simulink model "SHEV_Camaro_PwrLossMdl"  (R2018b)
settings: Solver=ode2  StartTime=0.0  StopTime=simDrv.time_s(end)  FixedStep=t_step  RelTol=1e-3
values from neighbouring files (symbols this model uses):
  A123_ESS =     [PwrLossMdl_A123Battery.mat]
  adj_motEffMap = [0.25 0.31 0.37 0.38 0.4 0.49 0.58 0.64 0.31 0.36 0.39 0.406 ... (72 elements, 8x9)]    [PwrLossMdl_PropSysEffData.mat]
  adjbsfc_map = [1051 1388 1174 1085 895 602 501 388 388 1051 1134 996 ... (81 elements, 9x9)]    [PwrLossMdl_GenSysEffData.mat]
  adjbsfc_spdbpt = [4003 4510 4987 5412 5800 5986 6322 6643 6889]    [PwrLossMdl_GenSysEffData.mat]
  adjbsfc_trqbpt = [10 15 20 25 30 35 40 45 50]    [PwrLossMdl_GenSysEffData.mat]
  C1 = [20000 20000 46318.5184323 46009.1793978 1021.23087801 1108.29786665 9922.48088723 10264.7269718 18293.5148586 29962.1621632 36298.3673472 37544.2700719 ... (41 elements, 1x41)]    [PwrLossMdl_ESS.mat]
  C2 = [20000 20000 46318.5184106 46009.1793608 1021.23035996 1108.29602087 9922.4809203 10264.72697 18293.5148606 29962.1621637 36298.3673482 37544.2700716 ... (41 elements, 1x41)]    [PwrLossMdl_ESS.mat]
  contMotTrq = [250 250 250 250 250 250 225 190 170]    [PwrLossMdl_PropSysEffData.mat]    (also in startPwrLossMdl.m = [180;180;180;180;180;180;180;180;170])
  cs_ll = 0.15    [startPwrLossMdl.m]
  cs_ul = 0.25    [startPwrLossMdl.m]
  E85_LHV = 30000    [startPwrLossMdl.m]
  mot_gbx_rat = 4.2    [startPwrLossMdl.m]
  motSpdVec = [1 500 1000 1500 2000 2500 3000 3500 4000]    [PwrLossMdl_PropSysEffData.mat]
  motTrqVec = [1 25 50 75 100 125 150 175]    [PwrLossMdl_PropSysEffData.mat]
  R0 = [0.5 0.5 0.413858741447 0.181330616185 0.123924684061 0.082623865753 0.114591066521 0.096554690516 0.0949331545326 0.124564294889 0.118490098825 0.107959033825 ... (41 elements, 1x41)]    [PwrLossMdl_ESS.mat]
  R1 = [0.5 0.5 0.513602817558 0.526624804767 0.484906164492 0.489343525408 0.493637128787 0.498122066152 0.500091294983 0.500054252951 0.500314275839 0.500483147312 ... (41 elements, 1x41)]    [PwrLossMdl_ESS.mat]
  R2 = [0.5 0.5 0.513602817535 0.526624804695 0.484906164494 0.489343525401 0.493637128787 0.498122066152 0.500091294984 0.50005425295 0.500314275838 0.500483147311 ... (41 elements, 1x41)]    [PwrLossMdl_ESS.mat]
  rho_fuel_gpL = 783    [startPwrLossMdl.m]
  simDrv = EEC_Single    [startPwrLossMdl.m]
  soc_bpt = [0 0.025 0.05 0.075 0.1 0.125 0.15 0.175 0.2 0.225 0.25 0.275 ... (41 elements, 1x41)]    [PwrLossMdl_ESS.mat]
  t_step = 0.1    [startPwrLossMdl.m]
  tire_rad_m = 0.346    [startPwrLossMdl.m]
  V_fuel_init_gal = 7    [startPwrLossMdl.m]
undefined symbols (not defined in the file or in its folder): DiscIntNeverNeededParam, N_OptResults, OptResults
libraries: simulink x10, custom_func x2, dspstat3 x1
(part 2 of 2)

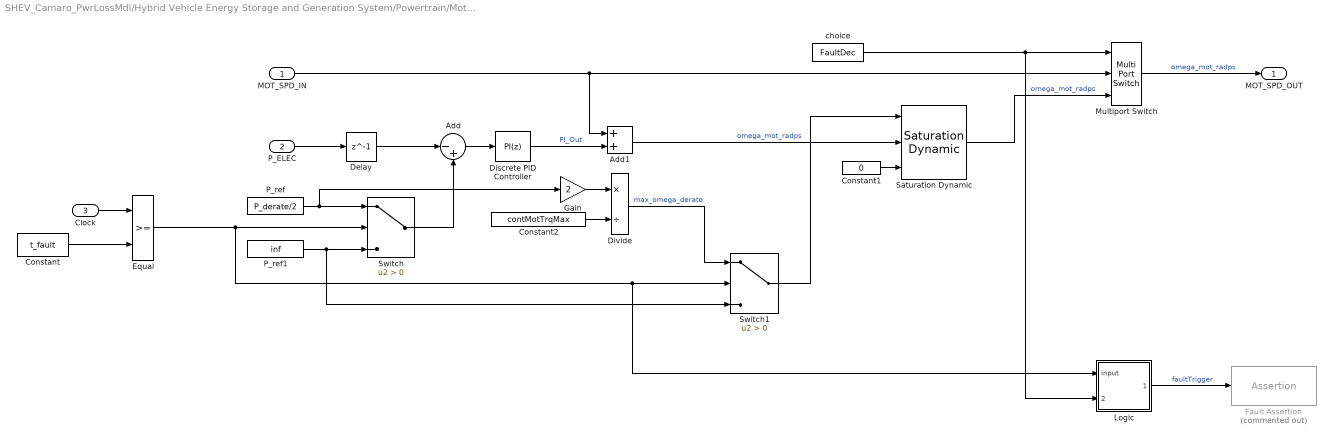
== system SHEV_Camaro_PwrLossMdl/Hybrid Vehicle Energy Storage and Generation System/Powertrain/Motor Fault Injection ==
  MOT_SPD_IN : Inport
  P_ELEC : Inport  Port=2
  Clock : Inport  Port=3
  Add : Sum  Inputs=|-+
  Add1 : Sum
  Constant : Constant  Value=t_fault
  Constant1 : Constant  Value=0
  Constant2 : Constant  Value=contMotTrqMax
  Delay : Delay  DelayLength=1
  Discrete PID Controller : simulink/Continuous/PID Controller  Controller=PI  Form=Parallel  TimeDomain=Discrete-time  SampleTime=-1  IntegratorMethod=Forward Euler  FilterMethod=Forward Euler  ControllerParametersSource=internal  P=0.002  I=0.003  D=0  UseFilter=on  N=100  TunerSelectOption=Transfer Function Based (PID Tuner App)  InitialConditionSource=internal  InitialConditionForIntegrator=0  InitialConditionForFilter=0  DifferentiatorICPrevScaledInput=0  ExternalReset=none  TrackingMode=off  Kt=1  LimitOutput=on  UpperSaturationLimit=0  LowerSaturationLimit=-inf  LinearizeAsGain=off  AntiWindupMode=clamping  Kb=1  POutMin=[]  POutMax=[]  IOutMin=[]  IOutMax=[]  DOutMin=[]  DOutMax=[]  NOutMin=[]  NOutMax=[]  SumOutMin=[]  SumOutMax=[]  SaturationOutMin=[]  SaturationOutMax=[]  PParamMin=[]  PParamMax=[]  IParamMin=[]  IParamMax=[]  DParamMin=[]  DParamMax=[]  NParamMin=[]  NParamMax=[]  KbParamMin=[]  KbParamMax=[]  KtParamMin=[]  KtParamMax=[]  KbOutMin=[]  KbOutMax=[]  KtOutMin=[]  KtOutMax=[]  IntegratorOutMin=[]  IntegratorOutMax=[]  FilterOutMin=[]  FilterOutMax=[]  SumI1OutMin=[]  SumI1OutMax=[]  SumI2OutMin=[]  SumI2OutMax=[]  SumI3OutMin=[]  SumI3OutMax=[]  SumI4OutMin=[]  SumI4OutMax=[]  SumDOutMin=[]  SumDOutMax=[]  DifferentiatorOutMin=[]  DifferentiatorOutMax=[]  FilterDiffOutCoefMin=[]  FilterDiffOutCoefMax=[]  ReciprocalOutMin=[]  ReciprocalOutMax=[]  SumDenOutMin=[]  SumDenOutMax=[]  SumNumOutMin=[]  SumNumOutMax=[]  DivideOutMin=[]  DivideOutMax=[]  IntegratorContinuousStateAttributes=''  IntegratorStateMustResolveToSignalObject=off  IntegratorRTWStateStorageClass=Auto  FilterContinuousStateAttributes=''  FilterStateMustResolveToSignalObject=off  FilterRTWStateStorageClass=Auto  ParallelPVariant=InternalParameters  IdealPVariant=Disabled  IVariant=InternalParameters  DVariant=Disabled  IntegratorVariant=Discrete  SatVariant=Enabled  AWVariant=DiscClampingParallel  PCopyVariant=Disabled  TRVariant=Disabled  FdbkBlocksVariant=Forward  IdealPFdbkVariant=Disabled  SatFdbkVariant=Disabled  DerivativeFilterVariant=Disabled  NVariant=Disabled  NCopyVariant=Disabled_SignalSpec  FilterICVariant=Disabled  IntegratorICVariant=InternalICs  ExternalResetVariant=Disabled  TRSumVariant=Passthrough  SumFdbkVariant=Disabled  SumVariant=Sum_PI
  Divide : Product  Inputs=*/
  Equal : RelationalOperator  OutDataTypeStr=boolean  RndMeth=Simplest
  Fault Assertion : Assertion  Commented=on  AssertionFailFcn=|  StopWhenAssertionFail=off
      | set_param(bdroot,'SimulationCommand','pause');
      | disp('## Paused due to Motor fault insertion')
  Gain : Gain  Gain=2
  Logic : Stateflow chart  TreatAsAtomicUnit=on
  Multiport Switch : MultiPortSwitch  DataPortOrder=Zero-based contiguous  Inputs=2  zeroidx=on
  P_ref : Constant  Value=P_derate/2
  P_ref1 : Constant  Value=inf
  Saturation Dynamic : simulink/Discontinuities/Saturation Dynamic  OutMin=[]  OutMax=[]  OutDataTypeStr=Inherit: Same as second input  OutDataType=fixdt(1, 16)  OutScaling=2^-10  DoSatur=off
  Switch : Switch  Criteria=u2 > Threshold
  Switch1 : Switch  Criteria=u2 > Threshold
  choice : Constant  Value=FaultDec
  MOT_SPD_OUT : Outport
  wires:
  Multiport Switch/1 -> MOT_SPD_OUT/1  "omega_mot_radps"
  choice/1 -> Logic/2(choice), Multiport Switch/1
  Add/1 -> Discrete PID Controller/1
  P_ELEC/1 -> Delay/1
  Delay/1 -> Add/1
  Discrete PID Controller/1 -> Add1/2  "PI_Out"
  MOT_SPD_IN/1 -> Multiport Switch/2, Add1/1
  P_ref/1 -> Gain/1, Switch/1
  Saturation Dynamic/1 -> Multiport Switch/3  "omega_mot_radps"
  Add1/1 -> Saturation Dynamic/2  "omega_mot_radps"
  Clock/1 -> Equal/1
  Constant/1 -> Equal/2
  Equal/1 -> Logic/1(input), Switch1/2, Switch/2
  Switch/1 -> Add/2
  P_ref1/1 -> Switch1/3, Switch/3
  Constant1/1 -> Saturation Dynamic/3
  Gain/1 -> Divide/1
  Constant2/1 -> Divide/2
  Divide/1 -> Switch1/1  "max_omega_derate"
  Switch1/1 -> Saturation Dynamic/1
  Logic/1(trigger) -> Fault Assertion/1  "faultTrigger"

== matlab function SHEV_Camaro_PwrLossMdl/Hybrid Vehicle Energy Storage and Generation System/Powertrain/MATLAB Function ==
  data: v_veh_mps input; v_veh_out_mps output; flag output
function [v_veh_out_mps,flag] = zerocheck(v_veh_mps)
    % Checks if the input speed is zero. 
    % If zero: sets the flag = 1, to change torque value to zero.
    % If not zero: sets the flag = 0, no change to the the torque value.
    
    if v_veh_mps == 0
        flag = 1;
        v_veh_out_mps = v_veh_mps;
    else
        flag = 0;
        v_veh_out_mps = v_veh_mps;
    end
end

== matlab function SHEV_Camaro_PwrLossMdl/Hybrid Vehicle Energy Storage and Generation System/MATLAB Function ==
  data: inp input; out output
function out = addnoise(inp)
snr = 25;

out = awgn(inp,snr,'measured');

== matlab function SHEV_Camaro_PwrLossMdl/Vehicle 2DOF Longitudinal and Pitch Model/Vehicle Dynamics Model 2 DOF (Longitudinal and Pitch) ==
  data: v_spd input; P_veh output; rg_pct input; dt input; Trq_dem output; acc_veh output; KE_veh output; Pwr_RR output; Pwr_Load output; dist_m output; elev_m output
function [P_veh, Trq_dem, acc_veh, KE_veh, Pwr_RR, Pwr_Load, dist_m, elev_m] = vehdyn2dof(v_spd,rg_pct,dt)
    % DESCRIPTION: The 2DOF Longitudinal and Pitch Model for the vehicle
    % uses the longitudinal road load equation comprising of Aerodynamic
    % Resistance, Climbing Resistance, Rolling Resistance as resistive
    % forces on the vehicle.
    %
    % F_veh [N] = F_trac + F_ar + F_cr + F_rr;  --------- (1)
    % P_veh [W] = F_veh [N] * v_veh [m/s];      --------- (2)
    %
    % Note: Pitch dynamics will be added to the model once COG height for
    % the car is determined. Currently only 1DOF longitudinal dynamics
    % exist.
    
    %% Pre-processing
    persistent v_spd_old dist elev
    if isempty(v_spd_old) && isempty(dist) && isempty(elev)
        v_spd_old = v_spd;
        dist = 0;
        elev = 0;
        flag = 1;
    else
        flag = 0;
    end
    alpha = atan(rg_pct/100);
    
    %% Static Parameters
    % -- Vehicle
    A_veh = 0.4;        % [m^2]
    C_d = 0.34;         % drag coefficient [-]
    m_veh = 2012;       %1875;       % [kg]
    P_tire = 32;        % [psi]
    R_tire = 0.346;     % [m]
    N_drvnWhl = 2;      % [-]
    Rat_gbx = 4.2;
    
    % -- Environment
    g = 9.81;           % acceleration due to gravity [m/s^2]
    rho_air = 1.225;    % STP density [kg/m^3]
    
    %% Dynamic Parameters
    C_rr = 0.005 + ((0.06895/P_tire) * ...
        (0.01 + (0.0095 * ((2.778 * (10^-3) * v_spd)^2))));            
    % function of tire pressure and vehicle speed [psi, mps]
    
    %% Vehicle Power Calculation
    if flag == 1
        P_veh = 0;
        Trq_dem = 0; 
        acc_veh = 0;
        KE_veh = 0;
        Pwr_RR = 0;
        Pwr_Load = 0;
        dist_m = dist;
        elev_m = elev;
    else
        acc_veh = (v_spd - v_spd_old)/dt;
        P_veh = ((m_veh * acc_veh) + ...
            (0.5 * rho_air * A_veh * C_d * (v_spd ^ 2)) + ...
            (m_veh * g * sin(alpha)) + ...
            (C_rr * m_veh * g)) * (v_spd);
        Trq_dem = ((P_veh/v_spd) * R_tire)/((N_drvnWhl * Rat_gbx));
        KE_veh = 0.5 * m_veh * ((v_spd^2) - (v_spd_old^2));
        dist_del = (v_spd_old * dt) + (0.5 * acc_veh * (dt^2));
        dist = dist + dist_del;
        elev = elev + ((rg_pct/100)*dist_del);
        dist_m = dist;
        elev_m = elev;
        v_spd_old = v_spd;
        Pwr_RR = (C_rr * m_veh * g) * (v_spd);
        Pwr_Load = ((0.5 * rho_air * A_veh * C_d * (v_spd ^ 2)) + ...
            (m_veh * g * sin(alpha)) + ...
            (C_rr * m_veh * g)) * (v_spd);
    end
    
end

== stateflow chart SHEV_Camaro_PwrLossMdl/Hybrid Vehicle Energy Management Control/Regen Braking Algorithm ==
  note: %P_reg_W
  state NoBraking
    du:
    P_reg_W = 0;
    P_mechbrk_W = 0;
    P_batt_W = P_elec_W;
  state Braking
    state RegenDisabled
      du:
      P_reg_W = 0;
      P_mechbrk_W = P_elec_W;
      P_batt_W = 0;
    state RegenEnabled
      state LightBraking
        du:
        P_reg_W = P_elec_W;
        P_mechbrk_W = P_elec_W - P_reg_W;
        P_batt_W = P_reg_W;
      state HeavyBraking
        du:
        P_reg_W = P_motreg_max_W;
        P_mechbrk_W = P_elec_W - P_reg_W;
        P_batt_W = P_reg_W;
      (default) -> LightBraking
      LightBraking -> HeavyBraking : [P_elec_W <= ...
          | P_motreg_max_W]
      HeavyBraking -> LightBraking : [P_elec_W >= ...
          | P_motreg_max_W]
    (default) -> RegenDisabled
    RegenDisabled -> RegenEnabled : [SoC <= 0.95]
    RegenEnabled -> RegenDisabled : [SoC > 0.95]
  (default) -> NoBraking
  NoBraking -> Braking : [P_elec_W < 0]
  Braking -> NoBraking : [P_elec_W >= 0]
  data: P_elec_W input; P_motreg_max_W input; P_mechbrk_W output double; P_batt_W output double; P_reg_W local double; SoC input

== stateflow chart SHEV_Camaro_PwrLossMdl/Hybrid Vehicle Energy Storage and Generation System/Battery EPO Logic/Battery EPO Constraint Logic ==
  state NoEPO
    du:
    epo_flag = 0;
  state EPO
    du:
    epo_flag = 1;
  (default) -> NoEPO
  NoEPO -> EPO : [LoadCurr < DchgCurrLim]
  EPO -> NoEPO : [LoadCurr >= DchgCurrLim]
  data: DchgCurrLim input; LoadCurr input; epo_flag output double

== stateflow chart SHEV_Camaro_PwrLossMdl/Hybrid Vehicle Energy Management Control/Rule Based Algorithm - Standard/Rule-Based Energy Mode Control ==
  state Initialization
  state CDMode
    du:
    mode = 0;
    genstat = 0;
  state CSModeGen
    du:
    mode = 1;
    genstat = 1;
  state CSModeNoGen
    du:
    mode = 1;
    genstat = 0;
  (default) -> Initialization
  Initialization -> (junction 7) [order 1] : [batsoc_frac <= init_soc && ...
      | batsoc_frac >= cs_ll]
  Initialization -> (junction 10) [order 2] : [batsoc_frac < cs_ll]
  (junction 7) -> CDMode
  (junction 10) -> CSModeGen
  CDMode -> CSModeGen : [batsoc_frac < cs_ll]
  CSModeGen -> CSModeNoGen : [batsoc_frac >= cs_ul]
  CSModeNoGen -> CSModeGen : [batsoc_frac < cs_ll]
  data: batsoc_frac input; cs_ll input; cs_ul input; init_soc input; genstat output double; mode output double

== matlab function SHEV_Camaro_PwrLossMdl/Hybrid Vehicle Energy Management Control/Rule Based Algorithm - Standard/Variable Power Request ==
  data: VehSpd_kph input; PwrMode output
function PwrMode = VarPwrReq(VehSpd_kph)
    if VehSpd_kph >= 0 && VehSpd_kph < 48
        PwrMode = 0;
    elseif VehSpd_kph >= 48 && VehSpd_kph < 97
        PwrMode = 1;
    else
        PwrMode = 2;
    end
end

== matlab function SHEV_Camaro_PwrLossMdl/Hybrid Vehicle Energy Storage and Generation System/A123 ESS Model/OCV_Battery/OCV Function ==
  data: soc input; ocv output; current input
function ocv = fcn(soc, current)

if current < 0
    %% 0-20 Model Fit
    if (soc <= 0.2)
        ocv = 3.17*exp(0.1*soc) - 2.76*exp(-65.25*soc);
    %% 20-80 Model Fit
    elseif (soc > 0.2 && soc <= 0.8)
        ocv = 0.155*soc + 3.2;
        % ocv = 0.165*soc + 3.20; OG
    %% 80-100 Model Fit
    else
        ocv = 0.2*(soc^74.2) + 3.33;
    end
else
    %% 0-20 Model Fit
    if (soc <= 0.2)
        ocv = 3.19*exp(0.098*soc) - 1.09*exp(-48.81*soc);
    %% 20-80 Model Fit
    elseif (soc > 0.2 && soc <= 0.8)
        ocv = 0.148*soc + 3.2;
        % ocv = 0.148*soc + 3.222;
    %% 80-100 Model Fit
    else
        ocv = 0.336*(soc^108.2) + 3.34;
    end
end

== stateflow chart SHEV_Camaro_PwrLossMdl/Hybrid Vehicle Energy Management Control/Proposed ReOpt DP Algorithm/Wait ==
  state Initialization
    en:
    Counter = 0;
    Trigger = 1;
  state InState
    du:
    Trigger = 1;
  state Wait1
  state Wait
  state OutState
    en:
    Trigger = 0;
    du:
    Trigger = 1;
    ex:
    Trigger = 1;
  (default) -> Initialization
  Initialization -> InState
  Wait1 -> InState : after(5.0,sec)
  Wait -> InState [order 1] : [ReOptReq == 0]
  InState -> Wait : [ReOptReq == 1]
  OutState -> Wait1 : [ReOptReq == 0]
  Wait -> OutState [order 2] : after(5.0,sec){Counter = Counter + 1;}
  data: ReOptReq input; Trigger output double; Counter output double

== stateflow chart SHEV_Camaro_PwrLossMdl/Hybrid Vehicle Energy Management Control/REx Fault Insertion Subsystem/Logic ==
  state NoFault
    en:
    trigger = 1;
    du:
    trigger = 1;
  state Fault
    en:
    trigger = 0;
    du:
    trigger = 1;
  (default) -> NoFault
  NoFault -> Fault : [input1 == 0 ||...
      | input2 == 0]
  data: trigger output double; input1 input; input2 input

== matlab function SHEV_Camaro_PwrLossMdl/Hybrid Vehicle Energy Management Control/Proposed ReOpt DP Algorithm/Optimal Pgen Lookup ==
  data: index input; element output; vector input
function element = idxLookup(index,vector)
% idxLookup is a custom function that returns element corresponding to
% index in a 1-D vector.
element = vector(index);
end

== matlab function SHEV_Camaro_PwrLossMdl/Hybrid Vehicle Energy Management Control/Proposed ReOpt DP Algorithm/Optimal SoC Lookup ==
  data: index input; element output; vector input
function element = idxLookup(index,vector)
% idxLookup is a custom function that returns element corresponding to
% index in a 1-D vector.
element = vector(index);
end

== matlab function SHEV_Camaro_PwrLossMdl/Hybrid Vehicle Energy Management Control/Proposed ReOpt DP Algorithm/Optimal EC_Wh_m ==
  data: index input; element output; vector input
function element = idxLookup(index,vector)
% idxLookup is a custom function that returns element corresponding to
% index in a 1-D vector.
element = vector(index);
end

== stateflow chart SHEV_Camaro_PwrLossMdl/Hybrid Vehicle Energy Storage and Generation System/Powertrain/Motor Fault Injection/Logic ==
  state NoFault
    en:
    trigger = 1;
    du:
    trigger = 1;
  state Fault
    en:
    trigger = 0;
    du:
    trigger = 1;
  (default) -> NoFault
  NoFault -> Fault : [input == 1 && ...
      | choice == 1]
  data: trigger output double; input input; choice input

== matlab function SHEV_Camaro_PwrLossMdl/Hybrid Vehicle Energy Management Control/EREV EM Custom MPC/Custom SOC MPC ==
  data: x_soc_k input; u_soc_ref_vec input size=[30 1]; x_soc_est_k_1 output size=[30 1] [0..1]; u_Paux_k_1 input; u_P_gen_k_1 input; u_est_spd_vec input size=[30 1]; u_est_acc_vec input size=[30 1]; md_grade_vec input size=[30 1]; estHorizon input; ctlHorizon input; Ts input; P_gen_opt output size=[30 1]; SOC_opt output size=[30 1]; status output; p output
function [x_soc_est_k_1,P_gen_opt,SOC_opt,status,p]  = soc_mpc(x_soc_k,u_soc_ref_vec,u_Paux_k_1,u_P_gen_k_1,u_est_spd_vec,u_est_acc_vec,md_grade_vec,estHorizon,ctlHorizon,Ts)
% ,b,H,f,A
%% Linearized Vehicle Power Model - UW EREV
m = 2012;
g = 9.81;
% Aerodynamic Drag Resistance Power Coefficient
Af = 0.4;
Cd = 0.34;
rho = 1.225;
A1 = 0.5 * Af * Cd * rho;
% Rolling Resistance Power Coefficient
Cr = 0.00502;
B1 = m * g * Cr;
% Climbing Resistance Power Coefficient
C1 = m * g;
% Battery information
Ebatt = 18900;

%% Estimation vector 
persistent soc_est_vec
if isempty(soc_est_vec)
    soc_est_vec = ones([estHorizon 1]);
end

%% Model based estimation
Pbatt = zeros([estHorizon 1]);
for k = 1:estHorizon
    Pbatt(k,1) = u_Paux_k_1 - u_P_gen_k_1 + (m * u_est_spd_vec(k,1) * u_est_acc_vec(k,1))...
            + (A1 * (u_est_spd_vec(k,1)^3)) + (B1 * u_est_spd_vec(k,1))...
            + (C1 * (md_grade_vec(k,1)/100) * u_est_spd_vec(k,1));
    if Pbatt(k,1) < -15000
        Pbatt(k,1) = -15000;
    end
    if k == 1
        soc_est_vec(k,1) = x_soc_k - ((Ts/(Ebatt * 3600)) * Pbatt(k,1));
    else
        soc_est_vec(k,1) = soc_est_vec(k-1,1) - ((Ts/(Ebatt * 3600)) * Pbatt(k,1));
    end
end
x_soc_est_k_1 = soc_est_vec;
%% Optimal Generator Power - mpcqpActiveSetSolver
p1 = 1;
p2 = 1e8;
k1 = 0.000141 * Ts;  % g/W; %Ts/(3600*18900);    
k2 = 1;
H = eye(ctlHorizon * 3);
for j = 1:(ctlHorizon * 3)  
    if mod(j,3) == 1
        H(j,:) = H(j,:) * (p1 * k1 * k1);
    elseif mod (j,3) == 2
        H(j,:) = H(j,:) * (p2 * k2 * k2);
    else
        H(j,:) = H(j,:) * p2 * (u_soc_ref_vec(j/3)^2);
    end
end
H = 2 * H;
[L,p] = chol(H,'lower');
Linv = inv(L);

f = zeros([ctlHorizon*3 1]);
f(2:3:end) = -2 * p2 * k2 * k2 * u_soc_ref_vec(1:ctlHorizon);

ineqVec_1 = [1 0 0;
            -1 0 0;
             0 1 0;
             0 -1 0];
ineqVec_3 = [1 0 0 1 0 0 1 0 0;
            -1 0 0 -1 0 0 -1 0 0;
             0 1 0 0 1 0 0 1 0;
             0 -1 0 0 -1 0 0 -1 0];
ineqVec_5 = [1 0 0 1 0 0 1 0 0 1 0 0 1 0 0;
            -1 0 0 -1 0 0 -1 0 0 -1 0 0 -1 0 0;
             0 1 0 0 1 0 0 1 0 0 1 0 0 1 0;
             0 -1 0 0 -1 0 0 -1 0 0 -1 0 0 -1 0];
ineqVec_10 = [1 0 0 1 0 0 1 0 0 1 0 0 1 0 0 1 0 0 1 0 0 1 0 0 1 0 0 1 0 0;
             -1 0 0 -1 0 0 -1 0 0 -1 0 0 -1 0 0 -1 0 0 -1 0 0 -1 0 0 -1 0 0 -1 0 0;
              0 1 0 0 1 0 0 1 0 0 1 0 0 1 0 0 1 0 0 1 0 0 1 0 0 1 0 0 1 0;
              0 -1 0 0 -1 0 0 -1 0 0 -1 0 0 -1 0 0 -1 0 0 -1 0 0 -1 0 0 -1 0 0 -1 0];
ineqVec_15 = [ineqVec_5 ineqVec_10];
ineqVec_20 = [ineqVec_10 ineqVec_10];
ineqVec_25 = [ineqVec_5 ineqVec_20];
ineqVec_30 = [ineqVec_15 ineqVec_15];
switch ctlHorizon
    case 1
        mult = 1;
        A = ineqVec_1;
        b = [0 * mult; -15000 * mult; sum(x_soc_est_k_1(1:mult,1)); -(sum(x_soc_est_k_1(1:mult,1)) + (((15000 * Ts)/(18900 * 3600))*mult))];
        Aeq = [-(Ts/(18900 * 3600)) 1 0];
        beq = sum(x_soc_est_k_1(1:mult,1));
    case 3
        mult = 3;
        A = ineqVec_3;
        b = [0 * mult; -15000 * mult; sum(x_soc_est_k_1(1:mult,1)); -(sum(x_soc_est_k_1(1:mult,1)) + (((15000 * Ts)/(18900 * 3600))*mult))];
        tmp_Aeq = [-(Ts/(18900 * 3600)) 1 0];
        Aeq = [tmp_Aeq tmp_Aeq tmp_Aeq];
        beq = sum(x_soc_est_k_1(1:mult,1));
    case 5
        mult = 5;
        A = ineqVec_5;
        b = [0 * mult; -15000 * mult; sum(x_soc_est_k_1(1:mult,1)); -(sum(x_soc_est_k_1(1:mult,1)) + (((15000 * Ts)/(18900 * 3600))*mult))];
        tmp_Aeq = [-(Ts/(18900 * 3600)) 1 0];
        Aeq = [tmp_Aeq tmp_Aeq tmp_Aeq tmp_Aeq tmp_Aeq];
        beq = sum(x_soc_est_k_1(1:mult,1));
    case 10
        mult = 10;
        A = ineqVec_10;
        b = [0 * mult; -15000 * mult; sum(x_soc_est_k_1(1:mult,1)); -(sum(x_soc_est_k_1(1:mult,1)) + (((15000 * Ts)/(18900 * 3600))*mult))];
        tmp_Aeq = [-(Ts/(18900 * 3600)) 1 0];
        Aeq = [tmp_Aeq tmp_Aeq tmp_Aeq tmp_Aeq tmp_Aeq tmp_Aeq tmp_Aeq tmp_Aeq tmp_Aeq tmp_Aeq];
        beq = sum(x_soc_est_k_1(1:mult,1));
    case 15
        mult = 15;
        A = ineqVec_15;
        b = [0 * mult; -15000 * mult; sum(x_soc_est_k_1(1:mult,1)); -(sum(x_soc_est_k_1(1:mult,1)) + (((15000 * Ts)/(18900 * 3600))*mult))];
        tmp_Aeq = [-(Ts/(18900 * 3600)) 1 0];
        Aeq = [tmp_Aeq tmp_Aeq tmp_Aeq tmp_Aeq tmp_Aeq tmp_Aeq tmp_Aeq tmp_Aeq tmp_Aeq tmp_Aeq tmp_Aeq tmp_Aeq tmp_Aeq tmp_Aeq tmp_Aeq];
        beq = sum(x_soc_est_k_1(1:mult,1));
    case 20
        mult = 20;
        A = ineqVec_20;
        b = [0 * mult; -15000 * mult; sum(x_soc_est_k_1(1:mult,1)); -(sum(x_soc_est_k_1(1:mult,1)) + (((15000 * Ts)/(18900 * 3600))*mult))];
        tmp_Aeq = [-(Ts/(18900 * 3600)) 1 0];
        Aeq = [tmp_Aeq tmp_Aeq tmp_Aeq tmp_Aeq tmp_Aeq tmp_Aeq tmp_Aeq tmp_Aeq tmp_Aeq tmp_Aeq tmp_Aeq tmp_Aeq tmp_Aeq tmp_Aeq tmp_Aeq tmp_Aeq tmp_Aeq tmp_Aeq tmp_Aeq tmp_Aeq];
        beq = sum(x_soc_est_k_1(1:mult,1));
    case 25
        mult = 25;
        A = ineqVec_25;
        b = [0 * mult; -15000 * mult; sum(x_soc_est_k_1(1:mult,1)); -(sum(x_soc_est_k_1(1:mult,1)) + (((15000 * Ts)/(18900 * 3600))*mult))];
        tmp_Aeq = [-(Ts/(18900 * 3600)) 1 0];
        Aeq = [tmp_Aeq tmp_Aeq tmp_Aeq tmp_Aeq tmp_Aeq tmp_Aeq tmp_Aeq tmp_Aeq tmp_Aeq tmp_Aeq tmp_Aeq tmp_Aeq tmp_Aeq tmp_Aeq tmp_Aeq tmp_Aeq tmp_Aeq tmp_Aeq tmp_Aeq tmp_Aeq tmp_Aeq tmp_Aeq tmp_Aeq tmp_Aeq tmp_Aeq];
        beq = sum(x_soc_est_k_1(1:mult,1));
    case 30
        mult = 30;
        A = ineqVec_30;
        b = [0 * mult; -15000 * mult; sum(x_soc_est_k_1(1:mult,1)); -(sum(x_soc_est_k_1(1:mult,1)) + (((15000 * Ts)/(18900 * 3600))*mult))];
        tmp_Aeq = [-(Ts/(18900 * 3600)) 1 0];
        Aeq = [tmp_Aeq tmp_Aeq tmp_Aeq tmp_Aeq tmp_Aeq tmp_Aeq tmp_Aeq tmp_Aeq tmp_Aeq tmp_Aeq tmp_Aeq tmp_Aeq tmp_Aeq tmp_Aeq tmp_Aeq tmp_Aeq tmp_Aeq tmp_Aeq tmp_Aeq tmp_Aeq tmp_Aeq tmp_Aeq tmp_Aeq tmp_Aeq tmp_Aeq tmp_Aeq tmp_Aeq tmp_Aeq tmp_Aeq tmp_Aeq];
        beq = sum(x_soc_est_k_1(1:mult,1));
    otherwise
        mult = 30;
        A = ineqVec_30;
        b = [0 * mult; -15000 * mult; sum(x_soc_est_k_1(1:mult,1)); -(sum(x_soc_est_k_1(1:mult,1)) + (((15000 * Ts)/(18900 * 3600))*mult))];
        tmp_Aeq = [-(Ts/(18900 * 3600)) 1 0];
        Aeq = [tmp_Aeq tmp_Aeq tmp_Aeq tmp_Aeq tmp_Aeq tmp_Aeq tmp_Aeq tmp_Aeq tmp_Aeq tmp_Aeq tmp_Aeq tmp_Aeq tmp_Aeq tmp_Aeq tmp_Aeq tmp_Aeq tmp_Aeq tmp_Aeq tmp_Aeq tmp_Aeq tmp_Aeq tmp_Aeq tmp_Aeq tmp_Aeq tmp_Aeq tmp_Aeq tmp_Aeq tmp_Aeq tmp_Aeq tmp_Aeq];
        beq = sum(x_soc_est_k_1(1:mult,1));
end

opt = mpcqpsolverOptions;

iA0 = false(size(b));

[x,status] = mpcqpsolver(Linv,f,A,b,Aeq,beq,iA0,opt);
P_gen_opt = x(1:3:end);
SOC_opt = x(2:3:end);
end

== matlab function SHEV_Camaro_PwrLossMdl/Hybrid Vehicle Energy Management Control/Prediction Vector Generator/Kinematic State Predictor ==
  data: inpvec_dist_m output size=[30 1]; vehSpd_mps input; vehAcc_mps2 input; distTrvld_m input; inpvec_vehSpd_mps output size=[30 1]; inpvec_vehAcc_ms2 output size=[30 1]; est_horizon_samples input; Ts input
function [inpvec_dist_m, inpvec_vehSpd_mps, inpvec_vehAcc_ms2]...
    = genkinest(vehSpd_mps, vehAcc_mps2, distTrvld_m, est_horizon_samples, Ts)

persistent v_old
if isempty(v_old)
    v_old = vehSpd_mps;
end

% Calculate vehicle acceleration at current time
veh_acc = vehAcc_mps2;

% Generate kinematic prediction vectors for est_horizon_samples
% The estimation horizon samples are based on 1 second time step
N = est_horizon_samples;
%% Linear Estimation - Not that good
% 1. Vehicle speed estimate for N (1 second) steps:
u = ones([N 1]) * vehSpd_mps;
a = eye(N) * veh_acc;
t = 1:1:N;
% --  Clamping values
tmp_vehSpd = u + (a*t');
tmp_vehAcc = diag(a);
tmp_vehAcc(tmp_vehSpd > 35.76) = 0;
tmp_vehAcc(tmp_vehSpd < 0) = 0;
tmp_vehSpd(tmp_vehSpd > 35.76) = 35.76;
tmp_vehSpd(tmp_vehSpd < 0) = 0;
inpvec_vehSpd_mps  = tmp_vehSpd;
inpvec_vehAcc_ms2 = tmp_vehAcc;

% 2. Vehicle distance estimate for N (1 second) steps:
uu = ones([N 1]) * vehSpd_mps;
temp_dist_m = (uu .* t') + (0.5 * tmp_vehAcc .* (t'.^2));
temp_dist_m(temp_dist_m < 0) = 0;
inpvec_dist_m = temp_dist_m + distTrvld_m;  % 

%% Speed limited - Exponential function estimation
% The upper and lower bounds on speed limit vary the acceleration values
% throughout the estimation horizon
% LL_SPD = 0;         % 0 mph
% UL_SPD = 35.8;      % 80 mph
% 
% if veh_acc >= 0
%     b_coeff = (4.95/(UL_SPD - LL_SPD)) * vehSpd_mps + 0.05;
% else
%     b_coeff = -(4.95/(UL_SPD - LL_SPD)) * vehSpd_mps + 5;
% end
% 
% a_coeff = veh_acc*2;
% 
% t_range = 1:1:N;
% 
% u = ones([N 1]) * vehSpd_mps;
% 
% for i = 2:N
%     u(i,1) = u(i-1,1) + (a_coeff * exp(-b_coeff * t_range(i)));
% end
% 
% inpvec_vehSpd_mps = u;
% inpvec_vehAcc_ms2 = (a_coeff * exp(-b_coeff * t_range'));
% inpvec_dist_m = distTrvld_m + cumsum(inpvec_vehSpd_mps);
end

== matlab function SHEV_Camaro_PwrLossMdl/Hybrid Vehicle Energy Management Control/Prediction Vector Generator/Optimal SoC Lookup ==
  data: index input size=[30 1]; element output size=[30 1]; vector input
function element = idxLookup(index,vector)
% idxLookup is a custom function that returns element corresponding to
% index in a 1-D vector.
element = vector(index);
end

== matlab function SHEV_Camaro_PwrLossMdl/Hybrid Vehicle Energy Management Control/Prediction Vector Generator/Road Grade Lookup ==
  data: index input size=[30 1]; element output size=[30 1]; vector input
function element = idxLookup(index,vector)
% idxLookup is a custom function that returns element corresponding to
% index in a 1-D vector.
element = vector(index);
end

== matlab function SHEV_Camaro_PwrLossMdl/Hybrid Vehicle Energy Management Control/Prediction Vector Generator/Vectorized Index Finder ==
  data: inpVector input; idx output size=[30 1]; queryElement input size=[30 1]; OUTOFRANGE_FLAG output
% This is a custom function block designed to determine the index of a
% search element in the available vector.
%
% ------------ Made by: Aman V. Kalia -----------------------------------
% ------------ University of Washington, Seattle ------------------------
% ------------ Made on: 12/04/2019 --------------------------------------
%
% Features:
% 1. It also handles edge cases where a direct find doesn't result in an 
% output. 
% 2. It throws a warning flag if the query SoC is out of range. Helpful in
% retriggering a recalculation.

function [idx,OUTOFRANGE_FLAG] = findidx(inpVector,queryElement)
    % Get the length of the queryElement vector
    q_len = length(queryElement);
    
    persistent int_idx
    if isempty(int_idx)
        int_idx = ones([q_len 1]);
    end
    
    if isempty(inpVector)
        idx = zeros([q_len 1]);
        OUTOFRANGE_FLAG = -1;
        error('Input vector cannot be empty.')
    else
        % Limit check - outer condition 
        % Check if entire prediction vector is in range
        OUTOFRANGE_FLAG = 0;
        for i = 1:q_len
            if (queryElement(i) >= min(inpVector)) && (queryElement(i) <= max(inpVector))
                OUTOFRANGE_FLAG = 0;
                temp_idx = find(inpVector == queryElement(i),1,'first');
                if ~isempty(temp_idx)
%                     idx = temp_idx(1);
                    int_idx(i) = temp_idx(1);
                else
                    u_idx = find(inpVector >= queryElement(i),1,'first');
                    l_idx = find(inpVector < queryElement(i),1,'last');
                    if abs(inpVector(l_idx) - queryElement(i)) < abs(inpVector(u_idx) - queryElement(i))
%                         idx = l_idx(1);
                        int_idx(i) = l_idx(1);
                    else
%                         idx = u_idx(1);
                        int_idx(i) = u_idx(1);
                    end
                end
            else
                if i ~= 1
                    OUTOFRANGE_FLAG = 0;
                    int_idx(i) = int_idx(i-1);
                else
                    OUTOFRANGE_FLAG = 1;
                    break;
                end
            end
        end
        idx = int_idx;
    end
end

== stateflow chart SHEV_Camaro_PwrLossMdl/Hybrid Vehicle Energy Management Control/ReOptimization Subsystem/Wait ==
  state Initialization
    en:
    Counter = 0;
    Trigger = 1;
  state InState
    du:
    Trigger = 1;
  state Wait1
  state Wait
  state OutState
    en:
    Trigger = 0;
    du:
    Trigger = 1;
    ex:
    Trigger = 1;
  (default) -> Initialization
  Initialization -> InState
  Wait1 -> InState : after(5.0,sec)
  Wait -> InState [order 1] : [ReOptReq == 0]
  InState -> Wait : [ReOptReq == 1]
  OutState -> Wait1 : [ReOptReq == 0]
  Wait -> OutState [order 2] : after(5.0,sec){Counter = Counter + 1;}
  data: ReOptReq input; Trigger output double; Counter output double
